simulink model "Second_Model_2026_Static_Target_Circ_Ship_WET"  (R2022b)
settings: Solver=VariableStepAuto  StartTime=0.0  StopTime=150  RelTol=1e-3
model workspace (MAT data in the model file):
  dt = 0.01
(part 2 of 2)

== matlab function Second_Model_2026_Static_Target_Circ_Ship_WET/RLS_algorithm/RLS_Dynamic ==
  data: x_i input; y_i input; beta_i input; est_x output; est_y output; exec_time output
function [est_x, est_y, exec_time] = RLS_Dynamic(x_i, y_i, beta_i) 
% RLS_Dynamic_Final
% Performs Recursive Least Squares (RLS) tracking for a moving target.
% Inputs:
%
%   x_i, y_i : Our Ship's Position (Self)
%   beta_i   : Noisy Angle Measurement (Radians)
% Outputs:
%   est_x, est_y : Estimated Target Position

% --- Persistent Memory ---
persistent P X_i lambda lambda_rate

% --- Timing Setup ---
exec_time = 0; 
coder.extrinsic('tic', 'toc'); 
tStart = tic; 

% --- Initialization (Runs once at t=0) ---
if isempty(P)
    % We set P to 10000 so the filter isn't "stubborn" at the start.
    % It allows the estimate to snap to the true position in short time.
    P = 10000 * eye(2);  
    
    % FIX 2: Tuned Forgetting Factor (Lambda)
    % We start with a lower lambda to learn quickly, then slowly increase it.
    lambda = 0.95; 
    
    % The 'Rate' controls how fast it hardens. 
    lambda_rate = 0.8; 
end

if isempty(X_i)
    X_i = zeros(2, 1);  % X vector initialization as a zero vector
end

% --- 1. Construct Pseudolinear Measurement ---
% Measurement Vector (phi) and Scalar (z)
% Model: -x*sin(beta) + y*cos(beta) = y_obs*cos(beta) - x_obs*sin(beta)
phi_i = [-sin(beta_i); cos(beta_i)];
z_i   = y_i * cos(beta_i) - x_i * sin(beta_i);

% --- 2. Calculate RLS Updates ---

% A. Estimation Error
e = z_i - phi_i' * X_i;

% B. Calculate Gain Vector (g_k)
% We use 3e-5 for R (Noise Variance) to scale the denominator correctly.
R_cov = 3e-5; 
denominator = (lambda * R_cov) + (phi_i' * P * phi_i);
g_k = (P * phi_i) / denominator;

% C. Update State Vector (Position Estimate)
X_i = X_i + g_k * e;

% D. Update Covariance Matrix (P)
P = (1 / lambda) * (P - g_k * phi_i' * P);

% Prevents numerical crashes over long simulations.
P = 0.5 * (P + P');

% --- 3. Update Lambda (Annealing with Safety Cap) ---
% Slowly increase lambda to smooth out the noise...
lambda = lambda_rate * lambda + (1 - lambda_rate);

if lambda > 0.9999999
    lambda = 0.9999999;
end

% --- Outputs ---
est_x = X_i(1);
est_y = X_i(2);
exec_time = toc(tStart); 
end

== matlab function Second_Model_2026_Static_Target_Circ_Ship_WET/Target_position/Calculating_different_positions/linear position ==
  data: x_i input; x_lin output; y_i input; v_x input; v_y input; t input; y_lin output
function [x_lin, y_lin] = lin_target_pos(x_i, y_i, v_x, v_y, t)
    % Calculate the linear position in the X direction
    % Formula: x(t) = x_initial + (velocity_x * time)
    x_lin = x_i + (v_x * t);

    % Calculate the linear position in the Y direction
    % Formula: y(t) = y_initial + (velocity_y * time)
    y_lin = y_i + (v_y * t);

== matlab function Second_Model_2026_Static_Target_Circ_Ship_WET/angle out of positions ==
  data: self_pos_x input; beta output; self_pos_y input; target_pos_x input; target_pos_y input
function beta = angle_beta_calc(self_pos_x, self_pos_y, target_pos_x, target_pos_y)

% Calculate relative position (target relative to self)
dx = target_pos_x - self_pos_x;   % delta x
dy = target_pos_y - self_pos_y;   % delta y

% Line-of-sight (bearing) angle beta from self to target
% atan2 returns angle in radians, from -pi to +pi
% Positive angle is counterclockwise from the positive x-axis
beta = atan2(dy, dx);

== matlab function Second_Model_2026_Static_Target_Circ_Ship_WET/unwrapping ==
  settings: updateMethod=DISCRETE
  data: beta input; beta_unwrapped output
function beta_unwrapped = angle_unwrapper(beta)
%#codegen

% Persistent variable to store previous unwrapped angle
persistent beta_prev;
if isempty(beta_prev)
    beta_prev = 0;  % initial value on first call
end

% Define threshold for detecting 2π jumps
threshold = pi;

% Compute angle difference
delta = beta - mod(beta_prev, 2*pi);

% Unwrap: detect jumps larger than π and correct by ±2π
if delta > threshold
    delta = delta - 2*pi;
elseif delta < -threshold
    delta = delta + 2*pi;
end

% Update unwrapped angle
beta_unwrapped = beta_prev + delta;

% Save for next step
beta_prev = beta_unwrapped;

end

== matlab function Second_Model_2026_Static_Target_Circ_Ship_WET/errors_and_display_rls/Distance_error_rls ==
  data: x_est input; pct_err_dist output; y_est input; x_tgt input; y_tgt input; ref_plus_10 output; ref_minus_10 output
function [pct_err_dist, ref_plus_10, ref_minus_10] = Distance_error_rls(x_est, y_est, x_tgt, y_tgt)
    % Inputs:
    %   x_est, y_est: Estimated position (from RLS)
    %   x_tgt, y_tgt: Real Target position
    
    % --- 1. Calculate Distances (Range) ---
    dist_est = sqrt(x_est^2 + y_est^2);
    dist_tgt = sqrt(x_tgt^2 + y_tgt^2);
    
    % Safety for division by zero
    if dist_tgt < 0.001
        dist_tgt = 0.001;
    end

    % --- 2. Calculate Percentage Error ---

    pos_err = sqrt((x_est - x_tgt)^2 + (y_est - y_tgt)^2);

    pct_err_dist = (pos_err / dist_tgt) * 100;
    
    % --- 3. Reference Lines (Constants) ---
    % Since the output is Percentage, the bounds are simply +10 and -10.
    ref_plus_10 = 10;
    ref_minus_10 = -10;
end

== matlab function Second_Model_2026_Static_Target_Circ_Ship_WET/errors_and_display_rls/Calculate_axis_errors ==
  data: x_est input; pct_err_x output; y_est input; x_tgt input; y_tgt input; pct_err_y output; sleeve_x_up output; sleeve_x_down output; sleeve_y_up output; sleeve_y_down output
function [pct_err_x, pct_err_y, sleeve_x_up, sleeve_x_down, sleeve_y_up, sleeve_y_down] = Calculate_axis_errors(x_est, y_est, x_tgt, y_tgt)
    % Inputs:
    %   x_est, y_est: Estimated position
    %   x_tgt, y_tgt: Real Target position

    % --- 1. Calculate Percentage Errors (Per Axis) ---
    % Useful for statistics: "What is my % error on X?"
    if abs(x_tgt) < 0.001, x_tgt = 0.001; end
    if abs(y_tgt) < 0.001, y_tgt = 0.001; end
    
    pct_err_x = ((x_est - x_tgt) / x_tgt) * 100;
    pct_err_y = ((y_est - y_tgt) / y_tgt) * 100;

    % --- 2. Calculate Sleeve Bounds (The "Tunnel") ---
    % Useful for Visualization: Plot 'x_est' against these two lines.
    
    % Calculate 10% margin based on absolute position
    margin_x = 0.1 * abs(x_tgt);
    margin_y = 0.1 * abs(y_tgt);
    
    % Define Upper and Lower walls of the tunnel
    sleeve_x_up   = x_tgt + margin_x; % Real X + 10%
    sleeve_x_down = x_tgt - margin_x; % Real X - 10%
    
    sleeve_y_up   = y_tgt + margin_y; % Real Y + 10%
    sleeve_y_down = y_tgt - margin_y; % Real Y - 10%
end
